simulink model "check_equilibrium_discrete"  (R2019b)
settings: Solver=VariableStepAuto  StartTime=0.0  StopTime=10  RelTol=1e-3
values from neighbouring files (symbols this model uses):
  h_02 = 10.53    [script_check_equilibrium_discrete.m]    (also in script_task_2_nonlinear_discrete.m)
  ue = [ue1; ue2]    [script_check_equilibrium_discrete.m]
  xe1 = (k_2*sqrt(xe2)/k_1)^2    [script_check_equilibrium_discrete.m]    (also in script_task_2_nonlinear_discrete.m = 1.5563)
  xe2 = 25.53    [script_check_equilibrium_discrete.m]    (also in script_task_2_nonlinear_discrete.m = 4.47)
  ye = 15    [script_check_equilibrium_discrete.m]
undefined symbols (not defined in the file or in its folder): A, B, C, D
settings Model: Creator=NicSch02  LastModifiedBy=NicSch02

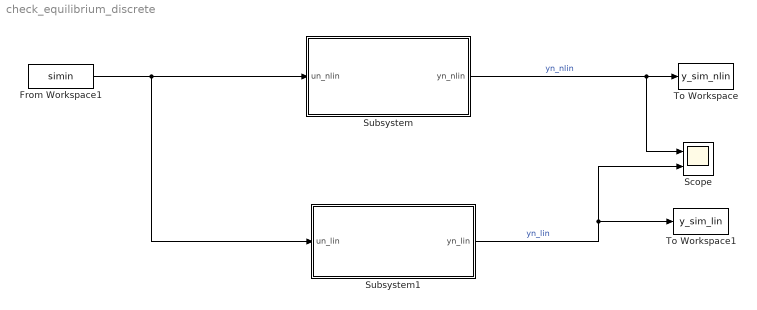
== system check_equilibrium_discrete ==
  From Workspace1 : FromWorkspace  VariableName=simin  SampleTime=0
  Scope : Scope  NumInputPorts=2
  Subsystem : Subsystem
  Subsystem1 : Subsystem
  To Workspace : ToWorkspace  VariableName=y_sim_nlin  SaveFormat=Structure With Time  SampleTime=-1
  To Workspace1 : ToWorkspace  VariableName=y_sim_lin  SaveFormat=Structure With Time  SampleTime=-1
  wires:
  From Workspace1/1 -> Subsystem1/1(un_lin), Subsystem/1(un_nlin)
  Subsystem/1(yn_nlin) -> Scope/1, To Workspace/1  "yn_nlin"
  Subsystem1/1(yn_lin) -> Scope/2, To Workspace1/1  "yn_lin"

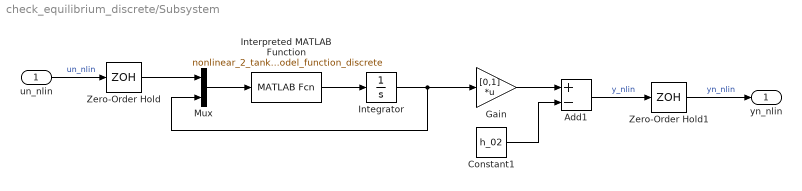
== system check_equilibrium_discrete/Subsystem ==
  un_nlin : Inport
  Add1 : Sum  Inputs=+-
  Constant1 : Constant  Value=h_02
  Gain : Gain  Gain=[0,1]  Multiplication=Matrix(K*u)
  Integrator : Integrator  InitialCondition=[xe1; xe2;]
  Interpreted MATLAB Function : MATLABFcn  MATLABFcn=nonlinear_2_tank_model_function_discrete
  Mux : Mux  Inputs=2
  Zero-Order Hold : ZeroOrderHold  SampleTime=0.5
  Zero-Order Hold1 : ZeroOrderHold  SampleTime=0.5
  yn_nlin : Outport
  wires:
  Integrator/1 -> Mux/2, Gain/1
  Constant1/1 -> Add1/2
  Interpreted MATLAB Function/1 -> Integrator/1
  Gain/1 -> Add1/1
  Mux/1 -> Interpreted MATLAB Function/1
  un_nlin/1 -> Zero-Order Hold/1  "un_nlin"
  Zero-Order Hold/1 -> Mux/1
  Add1/1 -> Zero-Order Hold1/1  "y_nlin"
  Zero-Order Hold1/1 -> yn_nlin/1  "yn_nlin"

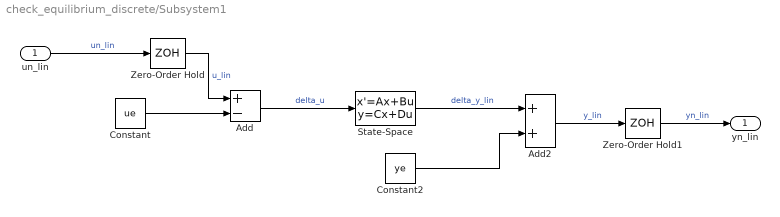
== system check_equilibrium_discrete/Subsystem1 ==
  un_lin : Inport
  Add : Sum  Inputs=+-
  Add2 : Sum
  Constant : Constant  Value=ue
  Constant2 : Constant  Value=ye
  State-Space : StateSpace  A=A  B=B  C=C  D=D  InitialCondition=[0; 0]
  Zero-Order Hold : ZeroOrderHold  SampleTime=0.5
  Zero-Order Hold1 : ZeroOrderHold  SampleTime=0.5
  yn_lin : Outport
  wires:
  Constant/1 -> Add/2
  Add/1 -> State-Space/1  "delta_u"
  Constant2/1 -> Add2/2
  State-Space/1 -> Add2/1  "delta_y_lin"
  un_lin/1 -> Zero-Order Hold/1  "un_lin"
  Zero-Order Hold/1 -> Add/1  "u_lin"
  Add2/1 -> Zero-Order Hold1/1  "y_lin"
  Zero-Order Hold1/1 -> yn_lin/1  "yn_lin"
